simulink model "W1P2"  (R2020b)
settings: Solver=VariableStepAuto  StartTime=0.0  StopTime=10.0  RelTol=1e-3
undefined symbols (not defined in the file): b, k1, k2, m1, m2
settings Model: Creator=Eshan  LastModifiedBy=Eshan

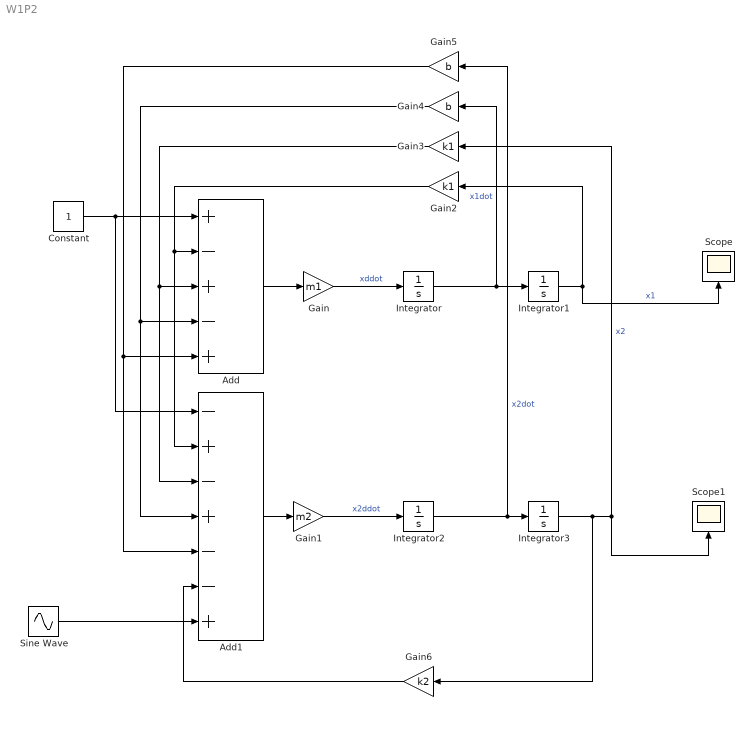
== system W1P2 ==
  Add : Sum  Inputs=+-+-+
  Add1 : Sum  Inputs=-+-+--+
  Constant : Constant
  Gain : Gain  Gain=m1
  Gain1 : Gain  Gain=m2
  Gain2 : Gain  Gain=k1
  Gain3 : Gain  Gain=k1
  Gain4 : Gain  Gain=b
  Gain5 : Gain  Gain=b
  Gain6 : Gain  Gain=k2
  Integrator{,1..3} (4 alike) : Integrator
  Scope : Scope
  Scope1 : Scope
  Sine Wave : Sin  Amplitude=k2  SampleTime=0
  wires:
  Gain6/1 -> Add1/6
  Sine Wave/1 -> Add1/7
  Gain4/1 -> Add1/4, Add/4
  Gain5/1 -> Add1/5, Add/5
  Gain3/1 -> Add1/3, Add/3
  Gain2/1 -> Add1/2, Add/2
  Integrator3/1 -> Gain6/1, Gain3/1, Scope1/1  "x2"
  Integrator/1 -> Gain4/1, Integrator1/1  "x1dot"
  Constant/1 -> Add1/1, Add/1
  Add/1 -> Gain/1
  Integrator1/1 -> Scope/1, Gain2/1  "x1"
  Gain/1 -> Integrator/1  "xddot"
  Add1/1 -> Gain1/1
  Gain1/1 -> Integrator2/1  "x2ddot"
  Integrator2/1 -> Gain5/1, Integrator3/1  "x2dot"
